simulink model "Uncertain_SAS_2_SubSystems"  (R2020a)
settings: Solver=VariableStepAuto  StartTime=0.0  StopTime=10.0  RelTol=1e-3
undefined symbols (not defined in the file): Asigma, bsigma, Csigma, Msigma, Nsigma
settings Model: Creator=d13go  LastModifiedBy=d13go

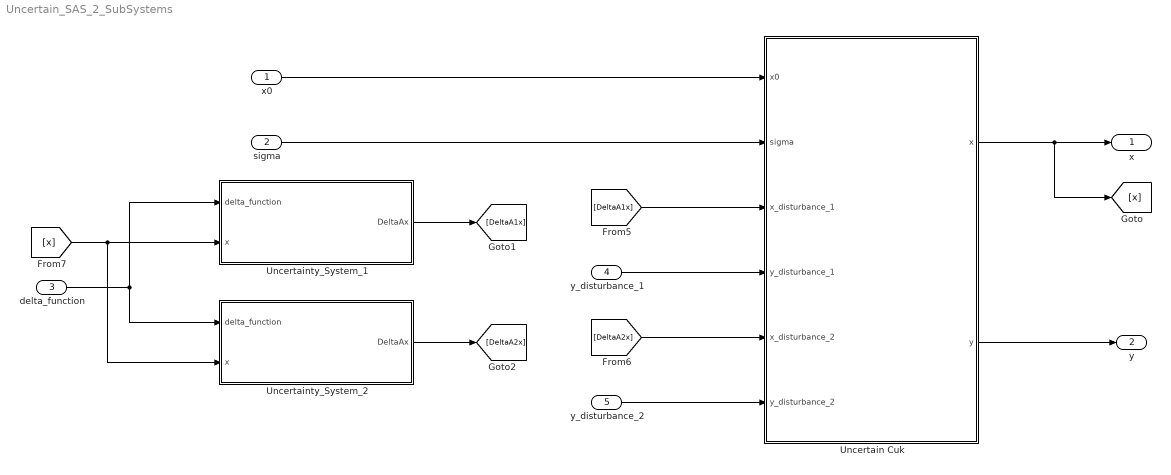
== system Uncertain_SAS_2_SubSystems ==
  x0 : Inport  PortDimensions=4
  sigma : Inport  Port=2
  delta_function : Inport  Port=3
  y_disturbance_1 : Inport  Port=4  PortDimensions=3
  y_disturbance_2 : Inport  Port=5  PortDimensions=3
  Uncertain Cuk : Subsystem  mask{A1=Asigma{1}, B1=bsigma{1}, C1=Csigma{1}, A2=Asigma{2}, B2=bsigma{2}, C2=Csigma{2}}
      mask prompts: A1 "Matrix A"; B1 "Matrix B"; C1 "Matrix C"; A2 "Matrix A"; B2 "Matrix B"; C2 "Matrix C"
      mask DialogControl DescTextVar Prompt: dx/dt = A(sigma)x+ b(sigma) + wx(sigma,x,u,t)
      mask DialogControl Control2 Prompt: y = C(sigma)x + wy(sigma,x,u,t)
      mask DialogControl Container3 Prompt: Subsystem 1
      mask DialogControl Container4 Prompt: Subsystem 2
      mask Display: disp('Switched Affine System State Space  \n with perturbations \n 2-Subsystems')
  Uncertainty_System_1 : Subsystem  mask{M=Msigma{1}, N=Nsigma{1}}
      mask prompts: M "M matrix"; N "N matrix"
      mask DialogControl DescTextVar Prompt: Uncertainties matrices of type \DeltaA = delta(t)*MaNa*x(t)
      mask Display: disp('Norm-bounded \n uncertainty')
  Uncertainty_System_2 : Subsystem  mask{M=Msigma{2}, N=Nsigma{2}}
      mask prompts: M "M matrix"; N "N matrix"
      mask DialogControl DescTextVar Prompt: Uncertainties matrices of type \DeltaA = delta(t)*MaNa*x(t)
      mask Display: disp('Norm-bounded \n uncertainty')
  x : Outport
  y : Outport  Port=2
  wires:
  Uncertainty_System_2/1(DeltaAx) -> [DeltaA2x]
  Uncertain Cuk/2(y) -> y/1
  Uncertain Cuk/1(x) -> [x], x/1
  [DeltaA1x] -> Uncertain Cuk/3(x_disturbance_1)
  Uncertainty_System_1/1(DeltaAx) -> [DeltaA1x]
  sigma/1 -> Uncertain Cuk/2(sigma)
  [x] -> Uncertainty_System_2/2(x), Uncertainty_System_1/2(x)
  delta_function/1 -> Uncertainty_System_1/1(delta_function), Uncertainty_System_2/1(delta_function)
  [DeltaA2x] -> Uncertain Cuk/5(x_disturbance_2)
  y_disturbance_2/1 -> Uncertain Cuk/6(y_disturbance_2)
  y_disturbance_1/1 -> Uncertain Cuk/4(y_disturbance_1)
  x0/1 -> Uncertain Cuk/1(x0)

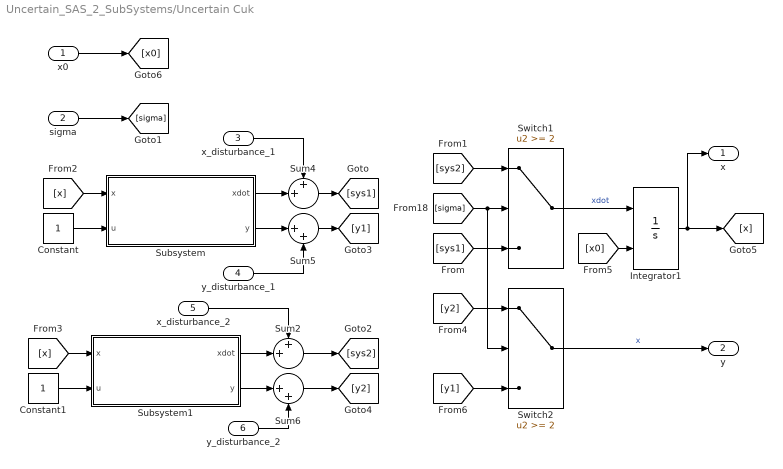
== system Uncertain_SAS_2_SubSystems/Uncertain Cuk ==
  x0 : Inport
  sigma : Inport  Port=2
  x_disturbance_1 : Inport  Port=3
  y_disturbance_1 : Inport  Port=4
  x_disturbance_2 : Inport  Port=5
  y_disturbance_2 : Inport  Port=6
  Constant : Constant
  Constant1 : Constant
  Integrator1 : Integrator  InitialConditionSource=external  InitialCondition=[0;0; 0; 0]
  Subsystem : Subsystem  mask{A=A1, B=B1, C=C1}
      mask prompts: A "Matrix A"; B "Matrix B"; C "Matrix C"
      mask Display: disp('Static State Space \n xdot = Ax+Bu\n y =Cx')
  Subsystem1 : Subsystem  mask{A=A2, B=B2, C=C2}
      mask prompts: A "Matrix A"; B "Matrix B"; C "Matrix C"
      mask Display: disp('Static State Space \n xdot = Ax+Bu\n y =Cx')
  Sum2 : Sum  Inputs=++|
  Sum4 : Sum  Inputs=++|
  Sum5 : Sum  Inputs=|++
  Sum6 : Sum  Inputs=|++
  Switch1 : Switch  Threshold=2
  Switch2 : Switch  Threshold=2
  x : Outport
  y : Outport  Port=2
  wires:
  [sys2] -> Switch1/1
  [sys1] -> Switch1/3
  [sigma] -> Switch2/2, Switch1/2
  Subsystem/1(xdot) -> Sum4/2
  Subsystem/2(y) -> Sum5/1
  Sum4/1 -> [sys1]
  Sum5/1 -> [y1]
  [x] -> Subsystem/1(x)
  Constant/1 -> Subsystem/2(u)
  Switch1/1 -> Integrator1/1  "xdot"
  [x0] -> Integrator1/2
  Integrator1/1 -> x/1, [x]
  Sum6/1 -> [y2]
  Sum2/1 -> [sys2]
  Subsystem1/2(y) -> Sum6/1
  [x] -> Subsystem1/1(x)
  Subsystem1/1(xdot) -> Sum2/2
  Constant1/1 -> Subsystem1/2(u)
  [y2] -> Switch2/1
  [y1] -> Switch2/3
  Switch2/1 -> y/1  "x"
  sigma/1 -> [sigma]
  x0/1 -> [x0]
  x_disturbance_1/1 -> Sum4/1
  y_disturbance_1/1 -> Sum5/2
  x_disturbance_2/1 -> Sum2/1
  y_disturbance_2/1 -> Sum6/2

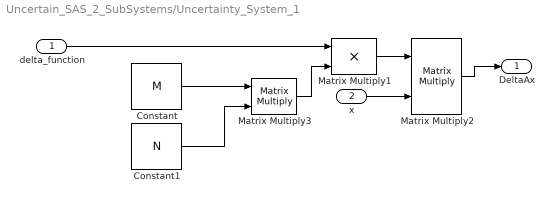
== system Uncertain_SAS_2_SubSystems/Uncertainty_System_1 ==
  delta_function : Inport
  x : Inport  Port=2
  Constant : Constant  Value=M
  Constant1 : Constant  Value=N
  Matrix Multiply1 : Product
  Matrix Multiply2 : Product  Multiplication=Matrix(*)
  Matrix Multiply3 : Product  Multiplication=Matrix(*)
  DeltaAx : Outport
  wires:
  Constant/1 -> Matrix Multiply3/1
  Constant1/1 -> Matrix Multiply3/2
  Matrix Multiply3/1 -> Matrix Multiply1/2
  delta_function/1 -> Matrix Multiply1/1
  Matrix Multiply1/1 -> Matrix Multiply2/1
  x/1 -> Matrix Multiply2/2
  Matrix Multiply2/1 -> DeltaAx/1

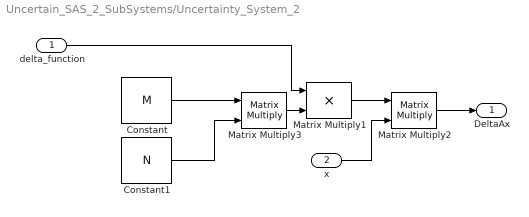
== system Uncertain_SAS_2_SubSystems/Uncertainty_System_2 ==
  delta_function : Inport
  x : Inport  Port=2
  Constant : Constant  Value=M
  Constant1 : Constant  Value=N
  Matrix Multiply1 : Product
  Matrix Multiply2 : Product  Multiplication=Matrix(*)
  Matrix Multiply3 : Product  Multiplication=Matrix(*)
  DeltaAx : Outport
  wires:
  Constant/1 -> Matrix Multiply3/1
  Constant1/1 -> Matrix Multiply3/2
  Matrix Multiply3/1 -> Matrix Multiply1/2
  delta_function/1 -> Matrix Multiply1/1
  Matrix Multiply1/1 -> Matrix Multiply2/1
  x/1 -> Matrix Multiply2/2
  Matrix Multiply2/1 -> DeltaAx/1

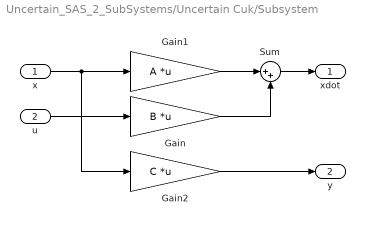
== system Uncertain_SAS_2_SubSystems/Uncertain Cuk/Subsystem ==
  x : Inport
  u : Inport  Port=2
  Gain : Gain  Gain=B  Multiplication=Matrix(K*u) (u vector)
  Gain1 : Gain  Gain=A  Multiplication=Matrix(K*u) (u vector)
  Gain2 : Gain  Gain=C  Multiplication=Matrix(K*u) (u vector)
  Sum : Sum  Inputs=|++
  xdot : Outport
  y : Outport  Port=2
  wires:
  u/1 -> Gain/1
  x/1 -> Gain2/1, Gain1/1
  Gain1/1 -> Sum/1
  Gain/1 -> Sum/2
  Sum/1 -> xdot/1
  Gain2/1 -> y/1

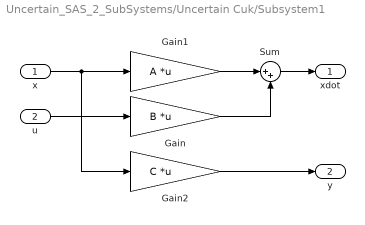
== system Uncertain_SAS_2_SubSystems/Uncertain Cuk/Subsystem1 ==
  x : Inport
  u : Inport  Port=2
  Gain : Gain  Gain=B  Multiplication=Matrix(K*u) (u vector)
  Gain1 : Gain  Gain=A  Multiplication=Matrix(K*u) (u vector)
  Gain2 : Gain  Gain=C  Multiplication=Matrix(K*u) (u vector)
  Sum : Sum  Inputs=|++
  xdot : Outport
  y : Outport  Port=2
  wires:
  u/1 -> Gain/1
  x/1 -> Gain2/1, Gain1/1
  Gain1/1 -> Sum/1
  Gain/1 -> Sum/2
  Sum/1 -> xdot/1
  Gain2/1 -> y/1
